simulink model "Mdl4ws_CS7"  (Simulink 7.0)
settings: Solver=ode45  SolverMode=SingleTasking  StartTime=0  StopTime=10  FixedStep=0.002  RelTol=1e-3  AbsTol=1e-6
libraries: Solver_SF x1
settings Model: Creator=dhall  LastModifiedBy=ywata  ExtModeTrigMode=oneshot  ExtModeArmWhenConnect=off
settings DataIOCC: LimitDataPoints=off  SignalLoggingName=sigsOut
settings OptimizationCC: BooleanDataType=off
settings DebuggingCC: SaveWithParameterizedLinksMsg=none  SignalResolutionControl=TryResolveAllWithWarning  SolverPrmCheckMsg=none  MultiTaskDSMMsg=warning  MultiTaskCondExecSysMsg=none  StrictBusMsg=None
settings HardwareCC: TargetUnknown=on
settings RTWCC: TemplateMakefile=grt_vc.tmf  IncludeERTFirstTime=on
settings GRTTargetCC: TargetFcnLib=ansi_tfl_tmw.mat  ModelReferenceCompliant=off  MatFileLogging=off

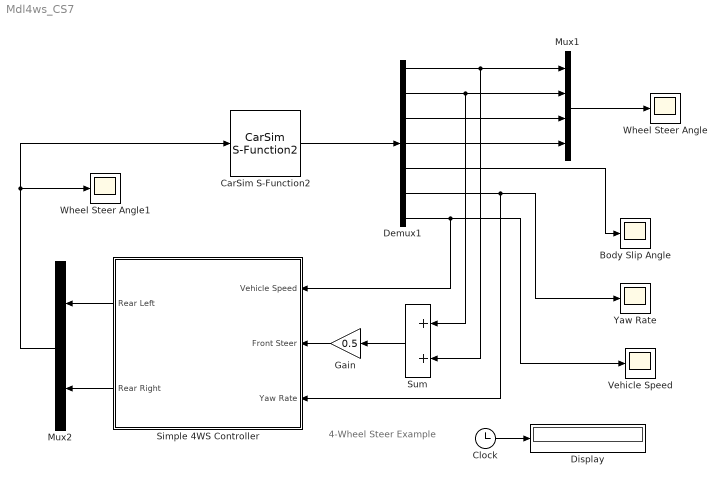
== system Mdl4ws_CS7 ==
  note: 4-Wheel Steer Example
  Body Slip Angle : Scope
      settings: TickLabels=on  YMin=-10  YMax=10  DataFormat=Array  Decimation=10
  CarSim S-Function2 : Solver_SF/CarSim S-Function2  Priority=1  VehicleCode=???
      settings: AttributesFormatString=Vehicle Code: %<VehicleCode>
  Clock : Clock
      settings: Decimation=10
  Demux1 : Demux  Outputs=[1 1 1 1 1 1 1]
  Display : Display
      settings: Format=bank  Decimation=100
  Gain : Gain  Orientation=left  Gain=0.5  ParameterDataType=sfix(16)  ParameterScaling=2^0  OutDataType=sfix(16)  OutScaling=2^0  SaturateOnIntegerOverflow=on
  Mux1 : Mux
  Mux2 : Mux  Orientation=left  Inputs=2
  Simple 4WS Controller : Subsystem  Orientation=left  mask{m=1530, lf=1.11, lr=1.666, Cf=97937, Cr=70287}
      mask prompts: m "body mass (kg)"; lf "length f-G (m)"; lr "length r-G (m)"; Cf "conering power f  (N/rad)"; Cr "conering power r  (N/rad)"
  Sum : Sum  Orientation=left  OutDataType=sfix(16)  OutScaling=2^0  SaturateOnIntegerOverflow=on  InputSameDT=on
  Vehicle Speed : Scope
      settings: TickLabels=on  YMin=0  YMax=150  DataFormat=Array  Decimation=10
  Wheel Steer Angle : Scope
      settings: TickLabels=on  YMin=-4  YMax=4  DataFormat=Array  Decimation=10
  Wheel Steer Angle1 : Scope
      settings: TickLabels=on  TimeRange=8  DataFormat=Array  Decimation=10
  Yaw Rate : Scope
      settings: TickLabels=on  YMin=-20  YMax=20  DataFormat=Array  Decimation=10
  wires:
  Sum/1 -> Gain/1
  Gain/1 -> Simple 4WS Controller/2(Front Steer)
  Mux1/1 -> Wheel Steer Angle/1
  Demux1/1 -> Sum/2, Mux1/1
  Demux1/2 -> Sum/1, Mux1/2
  Demux1/3 -> Mux1/3
  Demux1/4 -> Mux1/4
  Demux1/5 -> Body Slip Angle/1
  Demux1/6 -> Simple 4WS Controller/3(Yaw Rate), Yaw Rate/1
  Demux1/7 -> Simple 4WS Controller/1(Vehicle Speed), Vehicle Speed/1
  CarSim S-Function2/1 -> Demux1/1
  Simple 4WS Controller/1(Rear Left) -> Mux2/1
  Simple 4WS Controller/2(Rear Right) -> Mux2/2
  Clock/1 -> Display/1
  Mux2/1 -> Wheel Steer Angle1/1, CarSim S-Function2/1

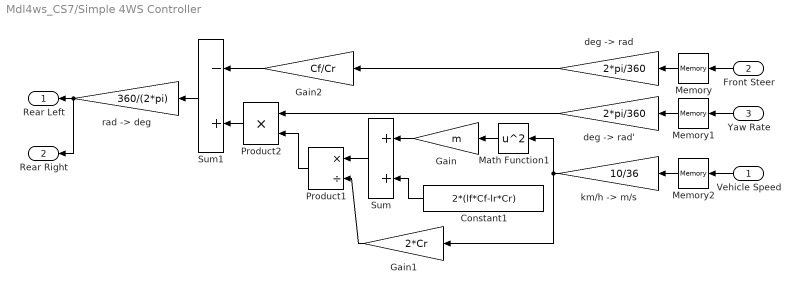
== system Mdl4ws_CS7/Simple 4WS Controller ==
  Vehicle Speed : Inport  Orientation=left  OutDataType=sfix(16)  OutScaling=2^0
  Front Steer : Inport  Orientation=left  Port=2  OutDataType=sfix(16)  OutScaling=2^0
  Yaw Rate : Inport  Orientation=left  Port=3  OutDataType=sfix(16)  OutScaling=2^0
  Constant1 : Constant  Orientation=left  Value=2*(lf*Cf-lr*Cr)  OutDataType=sfix(16)  OutScaling=2^0
  Gain : Gain  Orientation=left  Gain=m  ParameterDataType=sfix(16)  ParameterScaling=2^0  OutDataType=sfix(16)  OutScaling=2^0  SaturateOnIntegerOverflow=on
  Gain1 : Gain  Orientation=left  Gain=2*Cr  ParameterDataType=sfix(16)  ParameterScaling=2^0  OutDataType=sfix(16)  OutScaling=2^0  SaturateOnIntegerOverflow=on
  Gain2 : Gain  Orientation=left  Gain=Cf/Cr  ParameterDataType=sfix(16)  ParameterScaling=2^0  OutDataType=sfix(16)  OutScaling=2^0  SaturateOnIntegerOverflow=on
  Math Function1 : Math  Orientation=left  Operator=square  SaturateOnIntegerOverflow=on
  Memory : Memory  Orientation=left
  Memory1 : Memory  Orientation=left
  Memory2 : Memory  Orientation=left  X0=80
  Product1 : Product  Orientation=left  Inputs=*/  OutDataType=sfix(16)  OutScaling=2^0  SaturateOnIntegerOverflow=on  InputSameDT=on
  Product2 : Product  Orientation=left  OutDataType=sfix(16)  OutScaling=2^0  SaturateOnIntegerOverflow=on  InputSameDT=on
  Sum : Sum  Orientation=left  OutDataType=sfix(16)  OutScaling=2^0  SaturateOnIntegerOverflow=on  InputSameDT=on
  Sum1 : Sum  Orientation=left  Inputs=-+  OutDataType=sfix(16)  OutScaling=2^0  SaturateOnIntegerOverflow=on  InputSameDT=on
  "deg -> rad" : Gain  Orientation=left  Gain=2*pi/360  ParameterDataType=sfix(16)  ParameterScaling=2^0  OutDataType=sfix(16)  OutScaling=2^0  SaturateOnIntegerOverflow=on
  "deg -> rad'" : Gain  Orientation=left  Gain=2*pi/360  ParameterDataType=sfix(16)  ParameterScaling=2^0  OutDataType=sfix(16)  OutScaling=2^0  SaturateOnIntegerOverflow=on
  "km/h -> m/s" : Gain  Orientation=left  Gain=10/36  ParameterDataType=sfix(16)  ParameterScaling=2^0  OutDataType=sfix(16)  OutScaling=2^0  SaturateOnIntegerOverflow=on
  "rad -> deg" : Gain  Orientation=left  Gain=360/(2*pi)  ParameterDataType=sfix(16)  ParameterScaling=2^0  OutDataType=sfix(16)  OutScaling=2^0  SaturateOnIntegerOverflow=on
  Rear Left : Outport  Orientation=left  InitialOutput=0
  Rear Right : Outport  Orientation=left  Port=2  InitialOutput=0
  wires:
  Product1/1 -> Product2/2
  Product2/1 -> Sum1/2
  Gain1/1 -> Product1/2
  Constant1/1 -> Sum/2
  Math Function1/1 -> Gain/1
  Gain/1 -> Sum/1
  Sum/1 -> Product1/1
  Gain2/1 -> Sum1/1
  "km/h -> m/s"/1 -> Math Function1/1, Gain1/1
  "deg -> rad'"/1 -> Product2/1
  "deg -> rad"/1 -> Gain2/1
  Sum1/1 -> "rad -> deg"/1
  Front Steer/1 -> Memory/1
  Memory/1 -> "deg -> rad"/1
  Yaw Rate/1 -> Memory1/1
  Memory1/1 -> "deg -> rad'"/1
  Vehicle Speed/1 -> Memory2/1
  Memory2/1 -> "km/h -> m/s"/1
  "rad -> deg"/1 -> Rear Left/1, Rear Right/1
